simulink model "pedaling_distance"  (R2023a)
settings: Solver=VariableStepAuto  StartTime=0.0  StopTime=10.0  RelTol=1e-3
libraries: simulink x1
settings Model: Creator=hsllo  LastModifiedBy=hsllo

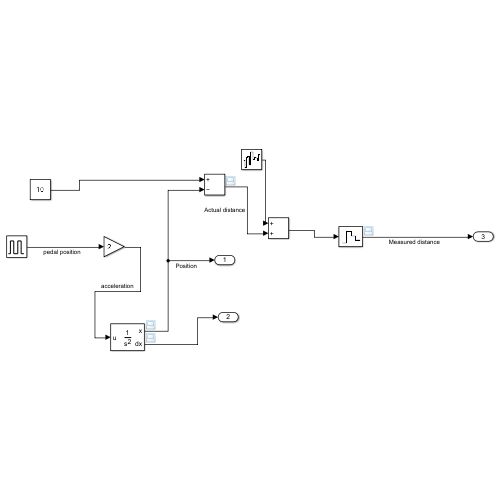
[thumbnail: Simulink's stored preview of the top-level diagram]
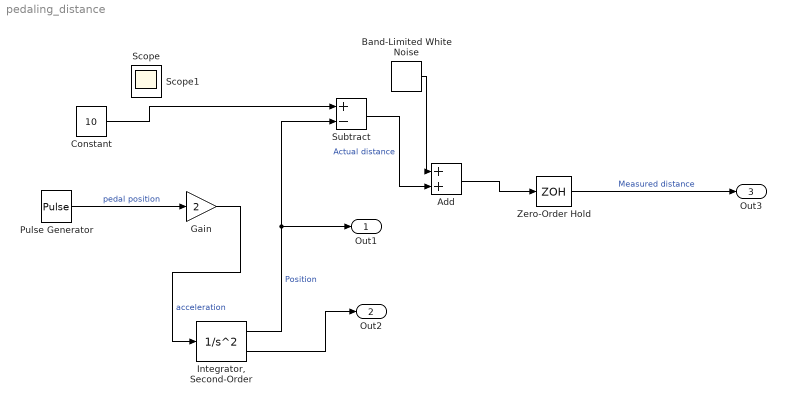
== system pedaling_distance ==
  Add : Sum
  Band-Limited White Noise : simulink/Sources/Band-Limited White Noise  Cov=[0.1]  Ts=0.1  seed=[23341]
  Constant : Constant  Value=10
  Gain : Gain  Gain=2
  "Integrator, Second-Order" : SecondOrderIntegrator
  Pulse Generator : DiscretePulseGenerator  PulseType=Time based  Period=10  PulseWidth=5
  Subtract : Sum  Inputs=+-
  Zero-Order Hold : ZeroOrderHold  SampleTime=-1
  Out1 : Outport
  Out2 : Outport  Port=2
  Out3 : Outport  Port=3
  Scope : Scope
  Scope1 : Scope
  wires:
  Pulse Generator/1 -> Gain/1  "pedal position"
  Gain/1 -> "Integrator, Second-Order"/1  "acceleration"
  "Integrator, Second-Order"/1 -> Subtract/2, Out1/1  "Position"
  "Integrator, Second-Order"/2 -> Out2/1
  Constant/1 -> Subtract/1
  Subtract/1 -> Add/2  "Actual distance"
  Band-Limited White Noise/1 -> Add/1
  Add/1 -> Zero-Order Hold/1
  Zero-Order Hold/1 -> Out3/1  "Measured distance"
